simulink model "Aula6_Simulink"  (R2013b)
settings: Solver=ode45  StartTime=0.0  StopTime=10.0  RelTol=1e-3
settings Model: Creator=ThiagoCordeiro  LastModifiedBy=ThiagoCordeiro

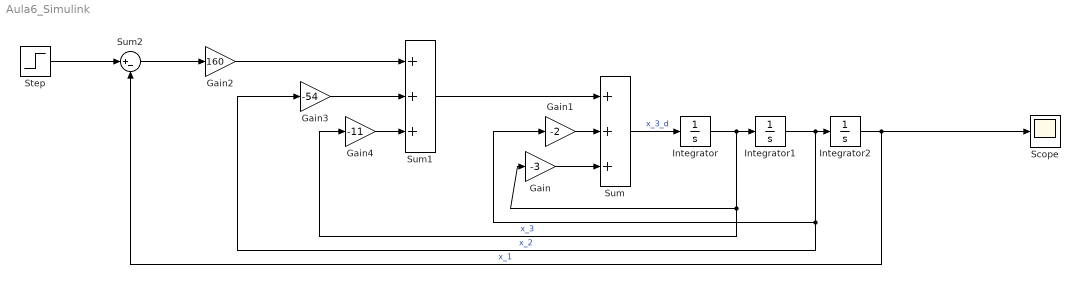
== system Aula6_Simulink ==
  Gain : Gain  Gain=-3
  Gain1 : Gain  Gain=-2
  Gain2 : Gain  Gain=160
  Gain3 : Gain  Gain=-54
  Gain4 : Gain  Gain=-11
  Integrator : Integrator
  Integrator1 : Integrator
  Integrator2 : Integrator
  Scope : Scope
  Step : Step  SampleTime=0
  Sum : Sum  Inputs=+++
  Sum1 : Sum  Inputs=+++
  Sum2 : Sum  Inputs=|+-
  wires:
  Integrator/1 -> Gain4/1, Gain/1, Integrator1/1  "x_3"
  Integrator1/1 -> Gain3/1, Gain1/1, Integrator2/1  "x_2"
  Integrator2/1 -> Sum2/2, Scope/1  "x_1"
  Gain/1 -> Sum/3
  Gain1/1 -> Sum/2
  Sum/1 -> Integrator/1  "x_3_d"
  Sum1/1 -> Sum/1
  Gain4/1 -> Sum1/3
  Gain3/1 -> Sum1/2
  Sum2/1 -> Gain2/1
  Gain2/1 -> Sum1/1
  Step/1 -> Sum2/1
